simulink library "Actuator_Lib"  (R2016b)
settings: Solver=ode45  StartTime=0.0  StopTime=10.0  RelTol=1e-3  EnableMultiTasking=on
undefined symbols (not defined in the file or in its folder): servo
undefined symbols (not defined in the file): AC
libraries: Actuator_Lib x2, simulink x1
settings Model: Creator=austinmurch  LastModifiedBy=katiekwiz
settings DataIOCC: LimitDataPoints=on  SaveFormat=Array  SignalLoggingSaveFormat=ModelDataLogs
settings OptimizationCC: ExpressionDepthLimit=2147483647  LifeSpan=inf  SimCompilerOptimization=on
settings DebuggingCC: UnderspecifiedInitializationDetection=Classic  MergeDetectMultiDrivingBlocksExec=none  SolverPrmCheckMsg=warning  FcnCallInpInsideContextMsg=warning  StateNameClashWarn=warning  StrictBusMsg=Warning  SFUnexpectedBacktrackingDiag=warning  SFNoUnconditionalDefaultTransitionDiag=warning  SFExecutionAtInitializationDiag=none
settings HardwareCC: ProdBitPerPointer=32  ProdBitPerSizeT=32  ProdBitPerPtrDiffT=32  ProdLargestAtomicFloat=None  ProdIntDivRoundTo=Undefined  ProdEndianess=Unspecified  ProdWordSize=32  ProdHWDeviceType=32-bit Generic
settings ModelReferenceCC: PropagateSignalLabelsOutOfModel=off
settings GRTTargetCC: TargetLangStandard=C89/C90 (ANSI)  GeneratePreprocessorConditionals=Disable all  CombineOutputUpdateFcns=off  GRTInterface=on
settings ConfigComp: CovMetricSettings=dw  CovHtmlReporting=on  CovSaveCumulativeToWorkspaceVar=on  CovSaveSingleToWorkspaceVar=on  CovExternalEMLEnable=off

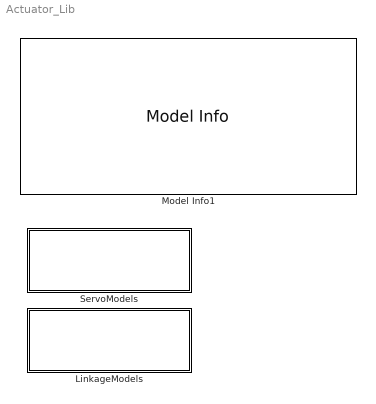
== system Actuator_Lib ==
  LinkageModels : Subsystem
  Model Info1 : simulink/Model-Wide Utilities/Model Info  BlockCM=None  Frame=on  DisplayStringWithTags=|  HorizontalTextAlignment=Left  LeftAlignmentValue=0.02  SourceBlockDiagram=Actuator_Lib  TagMaxNumber=20
      | MODEL INFORMATION
      | Actuator Model Library
      | 
      | University of Minnesota
      | Aerospace Engineering and Mechanics
      | Copyright 2011 Regents of the University of Minnesota. All rights reserved.
      | 
      | == SVN Info ==
      | Last modified by %<LastModifiedBy> on %<LastModificationDate>
  ServoModels : Subsystem

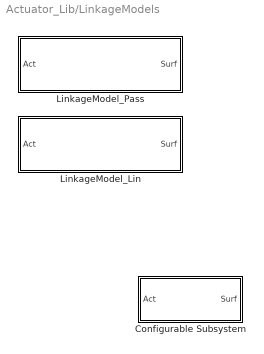
== system Actuator_Lib/LinkageModels ==
  Configurable Subsystem : Subsystem  BlockChoice=LinkageModel_Lin
      settings: TemplateBlock=self  MemberBlocks=LinkageModel_Lin,LinkageModel_Pass
  LinkageModel_Lin : Subsystem  VariantControl=VarLink_Lin  mask{link=AC.Surf}
      mask prompts: link "Linkage Structure:"
  LinkageModel_Pass : Subsystem  VariantControl=AC_TYPE_SIMPLE

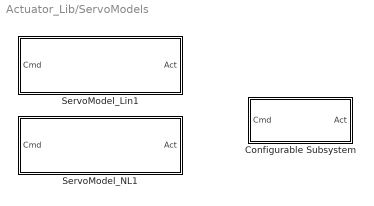
== system Actuator_Lib/ServoModels ==
  Configurable Subsystem : Subsystem  BlockChoice=ServoModel_Lin1
      settings: TemplateBlock=self  MemberBlocks=ServoModel_Lin1,ServoModel_NL1
  ServoModel_Lin1 : Subsystem  VariantControl=AC_TYPE_SIMPLE  mask(Rate and Position Limited Servo){act=servo}
      mask prompts: act "Actuator Structure"
      mask help: First order transfer function: w/(s+w), with rate and position limits.
      mask Help:
      | This block models a first order servo with the initial condition
      | on the integrator set to the steady state value for constant input.
      | The servo is rate and position limited and those values are set
      | in the block parameters.
  ServoModel_NL1 : Subsystem  VariantControl=VarServo_NL1  mask(Rate and Position Limited Servo){act=servo}
      mask prompts: act "Actuator Structure:"
      mask help: First order transfer function: w/(s+w), with rate and position limits.
      mask Help:
      | This block models a first order servo with the initial condition
      | on the integrator set to the steady state value for constant input.
      | The servo is rate and position limited and those values are set
      | in the block parameters.

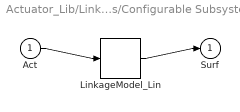
== system Actuator_Lib/LinkageModels/Configurable Subsystem ==
  Act : Inport
  LinkageModel_Lin : Actuator_Lib/LinkageModels/LinkageModel_Lin  VariantControl=VarLink_Lin  link=AC.Surf
  Surf : Outport
  wires:
  Act/1 -> LinkageModel_Lin/1
  LinkageModel_Lin/1 -> Surf/1

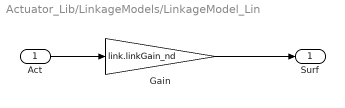
== system Actuator_Lib/LinkageModels/LinkageModel_Lin ==
  Act : Inport
  Gain : Gain  Gain=link.linkGain_nd
      settings: AttributesFormatString=%<Gain>
  Surf : Outport  PortDimensions=1
  wires:
  Act/1 -> Gain/1
  Gain/1 -> Surf/1

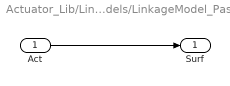
== system Actuator_Lib/LinkageModels/LinkageModel_Pass ==
  Act : Inport
  Surf : Outport  PortDimensions=1
  wires:
  Act/1 -> Surf/1

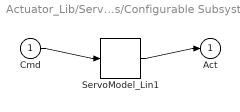
== system Actuator_Lib/ServoModels/Configurable Subsystem ==
  Cmd : Inport
  ServoModel_Lin1 : Actuator_Lib/ServoModels/ServoModel_Lin1  VariantControl=AC_TYPE_SIMPLE  act=servo
  Act : Outport
  wires:
  Cmd/1 -> ServoModel_Lin1/1
  ServoModel_Lin1/1 -> Act/1

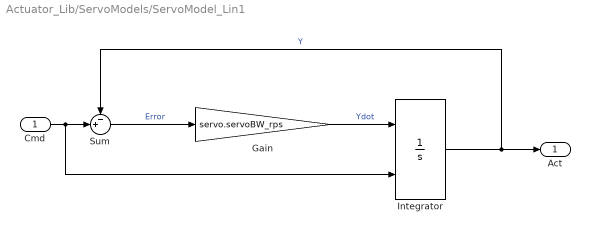
== system Actuator_Lib/ServoModels/ServoModel_Lin1 ==
  Cmd : Inport
  Gain : Gain  Gain=servo.servoBW_rps  SaturateOnIntegerOverflow=on  OutDataTypeStr=Inherit: Same as input  ParamDataTypeStr=Inherit: Same as input
  Integrator : Integrator  InitialConditionSource=external  UpperSaturationLimit=Inf  LowerSaturationLimit=-Inf  IgnoreLimit=on
  Sum : Sum  Inputs=-+|  SaturateOnIntegerOverflow=on  InputSameDT=on  OutDataTypeStr=Inherit: Same as first input
  Act : Outport  PortDimensions=1
  wires:
  Gain/1 -> Integrator/1  "Ydot"
  Sum/1 -> Gain/1  "Error"
  Integrator/1 -> Sum/1, Act/1  "Y"
  Cmd/1 -> Integrator/2, Sum/2

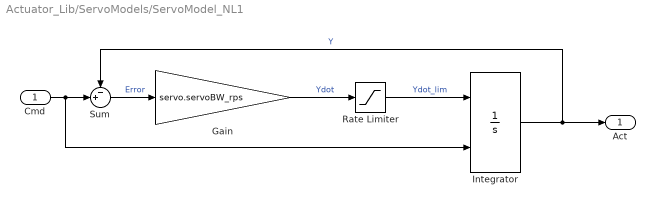
== system Actuator_Lib/ServoModels/ServoModel_NL1 ==
  Cmd : Inport
  Gain : Gain  Gain=servo.servoBW_rps  SaturateOnIntegerOverflow=on  OutDataTypeStr=Inherit: Same as input  ParamDataTypeStr=Inherit: Same as input
  Integrator : Integrator  InitialConditionSource=external  LimitOutput=on  UpperSaturationLimit=servo.servoLimPos_rad  LowerSaturationLimit=servo.servoLimNeg_rad  IgnoreLimit=on
  Rate Limiter : Saturate  UpperLimit=servo.servoRateLim_rps  LowerLimit=-servo.servoRateLim_rps
  Sum : Sum  Inputs=-+|  SaturateOnIntegerOverflow=on  InputSameDT=on  OutDataTypeStr=Inherit: Same as first input
  Act : Outport  PortDimensions=1
  wires:
  Cmd/1 -> Sum/2, Integrator/2
  Rate Limiter/1 -> Integrator/1  "Ydot_lim"
  Integrator/1 -> Act/1, Sum/1  "Y"
  Sum/1 -> Gain/1  "Error"
  Gain/1 -> Rate Limiter/1  "Ydot"
